simulink model "Ctrl_only"  (R2024a)
settings: Solver=FixedStepDiscrete  StartTime=0.0  StopTime=Inf  FixedStep=0.005  RelTol=1e-3
StopFcn:
  | user_confirmed = true;
  | disp('Gestoppt?!')
  | 
  | % stop(t);
  | % delete(t);
  | 
  | %% Switch to Config Mode
  | %Tc3_AI.sysManager.ActivateConfiguration();
  | %
  | % Tc3_AI.SwitchToConfig('local')
  | %
  | % %save Solution
  | % Tc3_AI.SaveSolution();
  | %
  | % %% Close Aktive VS Instance
  | % Tc3_AI.closeVsInstance();
libraries: slpidlib x1
settings Model: SimulationMode=external  Creator=clemensm  LastModifiedBy=pikronthaler
settings OptimizationCC: LocalBlockOutputs=off
settings RTWCC: Description=TwinCAT GRT Target  SystemTargetFile=TwinCatGrt.tlc  GenCodeOnly=on  GenerateMakefile=off  TemplateMakefile=tcgrt_msbuild.tmf  TargetLang=C++
settings STFCustomTargetCC: TargetLangStandard=C++11 (ISO)  ConcurrentExecutionCompliant=on  CombineOutputUpdateFcns=on  CodeInterfacePackaging=Reusable function  CPPClassGenCompliant=on  GRTInterface=off  GenerateAllocFcn=on  UseToolchainInfoCompliant=off  SystemTargetFile=TwinCatGrt.tlc
settings GRTTargetCC: TargetLangStandard=C++11 (ISO)  ParMdlRefBuildCompliant=off  CompOptLevelCompliant=off  MatFileLogging=off  CodeInterfacePackaging=Reusable function  GenerateAllocFcn=on  UseToolchainInfoCompliant=off  ExtMode=on  ExtModeMexFile=TcExtModeClient  MultiInstanceErrorCode=None

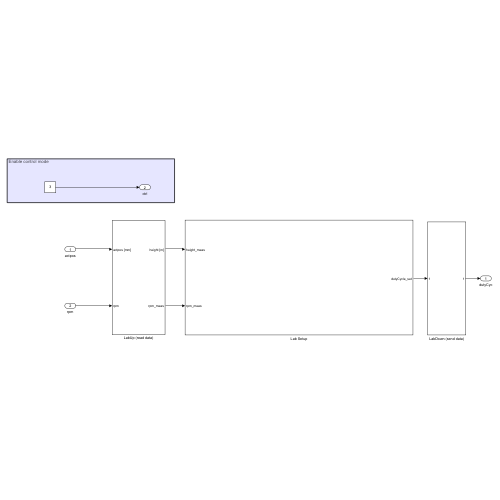
[thumbnail: Simulink's stored preview of the top-level diagram]
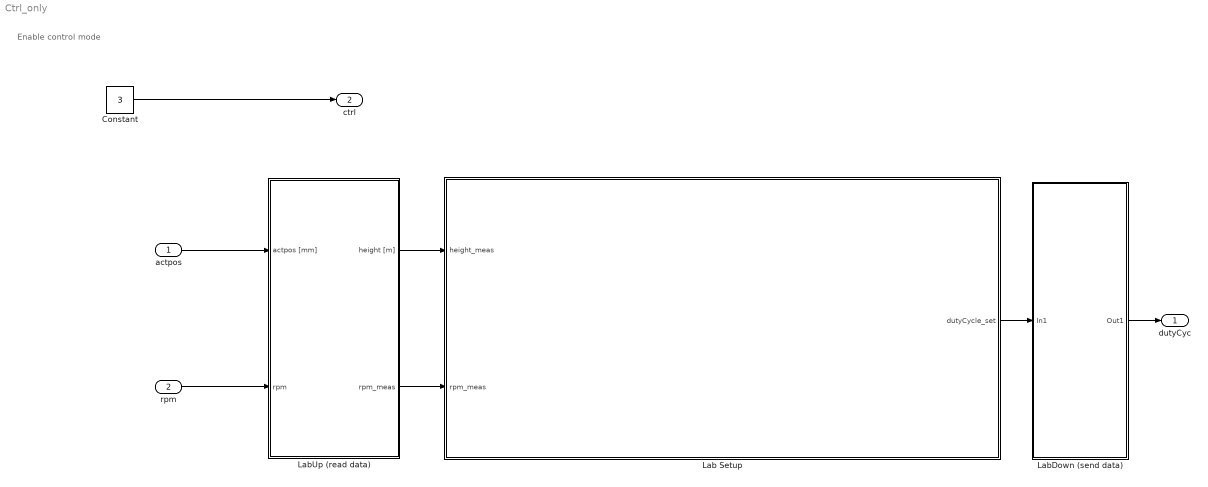
== system Ctrl_only ==
  note: Enable control mode
  actpos : Inport  OutDataTypeStr=uint16
  rpm : Inport  Port=2  OutDataTypeStr=uint16
  Constant : Constant  Value=3  OutDataTypeStr=uint8
  Lab Setup : Subsystem
  LabDown (send data) : Subsystem
  LabUp (read data) : Subsystem
  dutyCyc : Outport  OutDataTypeStr=uint16
  ctrl : Outport  Port=2  OutDataTypeStr=uint8
  wires:
  Constant/1 -> ctrl/1
  LabUp (read data)/2(rpm_meas) -> Lab Setup/2(rpm_meas)
  rpm/1 -> LabUp (read data)/2(rpm)
  LabUp (read data)/1(height [m]) -> Lab Setup/1(height_meas)
  actpos/1 -> LabUp (read data)/1(actpos [mm])
  Lab Setup/1(dutyCycle_set) -> LabDown (send data)/1(In1)
  LabDown (send data)/1(Out1) -> dutyCyc/1

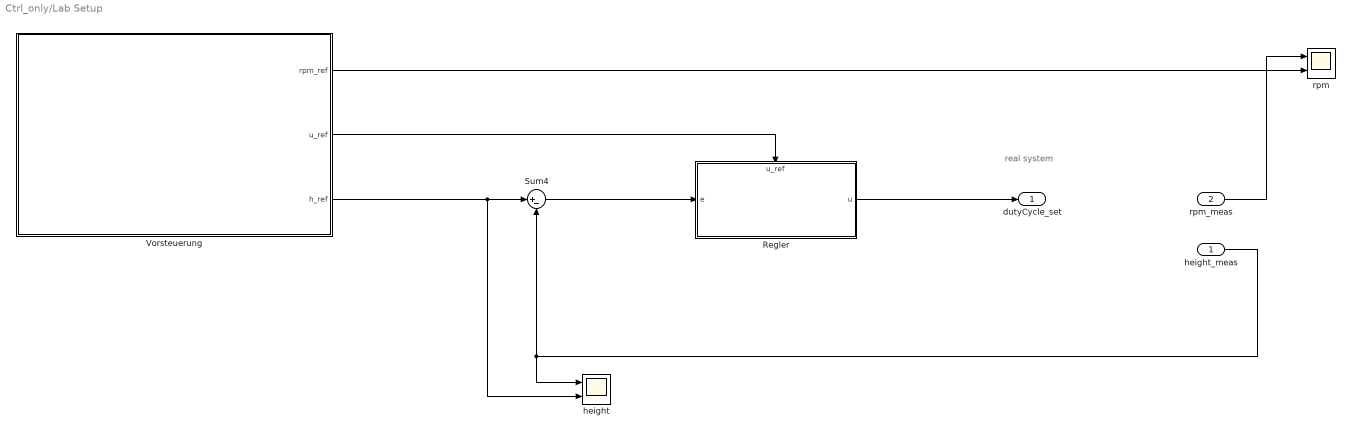
== system Ctrl_only/Lab Setup ==
  note: real system
  height_meas : Inport
  rpm_meas : Inport  Port=2
  Regler : Subsystem
      settings: PortSchema="{\"entries\":[{\"content\":{\"sides\":[{\"content\":{\"connectorIds\":[\"In1\"]},\"type\":\"ConnectorPlacement.EquallySpacedRectSide\",\"uuid\":\"368b1d1f-ffb1-4e6b-b9fe-083329fa83ff\"},{\"content\":{\"connectorIds\":[\"Out1\"],\"side\":\"RIGHT\"},\"type\":\"ConnectorPlacement.EquallySpacedRectSide\",\"uuid\":\"b6a3e5b0-4217-4560-ab72-51db08b1fa5c\"},{\"content\":{\"connectorIds\":[\"In2\"],\"side\":\"TOP\"},\"type\":\"ConnectorPlacement.EquallySpacedRectSide\",\"uuid\":\"ca46bd49-adac-4614-8e8d-04b2e9e52b66\"}]},\"type\":\"ConnectorPlacement.EquallySpacedConnector\",\"uuid\":\"bc9435da-4a52-4305-8584-3547e54afaf1\"}],\"packageUris\":[\"http://schema.mathworks.com/mf0/Connector/R2020b\"],\"version\":\"1.0\"}"
  Sum4 : Sum  Inputs=|+-
  Vorsteuerung : Subsystem
  height : Scope  NumInputPorts=2
  rpm : Scope  NumInputPorts=2
  dutyCycle_set : Outport
  wires:
  height_meas/1 -> Sum4/2, height/1
  rpm_meas/1 -> rpm/1
  Vorsteuerung/3(h_ref) -> height/2, Sum4/1
  Vorsteuerung/1(rpm_ref) -> rpm/2
  Vorsteuerung/2(u_ref) -> Regler/2(u_ref)
  Sum4/1 -> Regler/1(e)
  Regler/1(u) -> dutyCycle_set/1

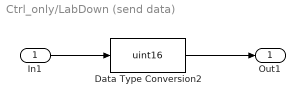
== system Ctrl_only/LabDown (send data) ==
  In1 : Inport
  Data Type Conversion2 : DataTypeConversion  OutDataTypeStr=uint16  SaturateOnIntegerOverflow=off  RndMeth=Floor
  Out1 : Outport
  wires:
  Data Type Conversion2/1 -> Out1/1
  In1/1 -> Data Type Conversion2/1

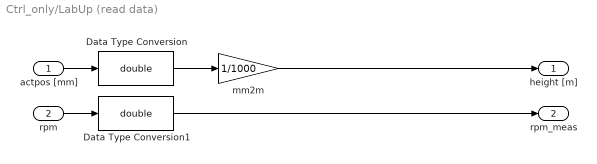
== system Ctrl_only/LabUp (read data) ==
  actpos [mm] : Inport  OutDataTypeStr=uint16
  rpm : Inport  Port=2
  Data Type Conversion : DataTypeConversion  OutDataTypeStr=double  SaturateOnIntegerOverflow=off  RndMeth=Floor
  Data Type Conversion1 : DataTypeConversion  OutDataTypeStr=double  SaturateOnIntegerOverflow=off  RndMeth=Floor
  mm2m : Gain  Gain=1/1000
  height [m] : Outport
  rpm_meas : Outport  Port=2
  wires:
  actpos [mm]/1 -> Data Type Conversion/1
  Data Type Conversion/1 -> mm2m/1
  mm2m/1 -> height [m]/1
  rpm/1 -> Data Type Conversion1/1
  Data Type Conversion1/1 -> rpm_meas/1

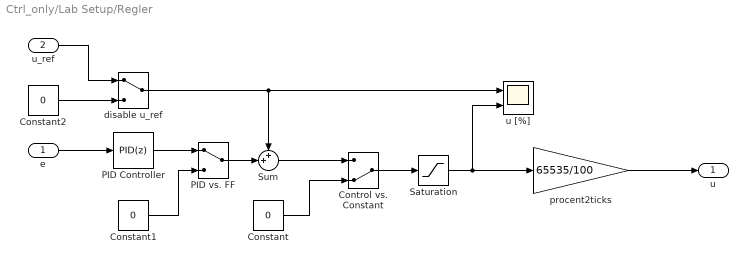
== system Ctrl_only/Lab Setup/Regler ==
  e : Inport
  u_ref : Inport  Port=2
  Constant : Constant  Value=0
  Constant1 : Constant  Value=0
  Constant2 : Constant  Value=0
  Control vs. Constant : ManualSwitch  CurrentSetting=0
  PID Controller : slpidlib/PID Controller  Controller=PID  Form=Parallel  TimeDomain=Discrete-time  UseExternalTs=off  SampleTime=-1  IntegratorMethod=Forward Euler  FilterMethod=Forward Euler  ControllerParametersSource=internal  P=1  I=1  UseKiTs=off  D=0  UseExternalDerivativeSource=off  N=100  UseFilter=on  TunerSelectOption=Transfer Function Based (PID Tuner App)  InitialConditionSource=internal  InitialConditionForIntegrator=0  InitialConditionForFilter=0  DifferentiatorICPrevScaledInput=0  ExternalReset=none  TrackingMode=off  Kt=1  LimitOutput=off  SatLimitsSource=internal  UpperSaturationLimit=inf  LowerSaturationLimit=-inf  LinearizeAsGain=on  AntiWindupMode=none  Kb=1  LimitIntegrator=off  UpperIntegratorSaturationLimit=inf  LowerIntegratorSaturationLimit=-inf  POutMin=[]  POutMax=[]  IOutMin=[]  IOutMax=[]  DOutMin=[]  DOutMax=[]  NOutMin=[]  NOutMax=[]  SumOutMin=[]  SumOutMax=[]  SaturationOutMin=[]  SaturationOutMax=[]  PParamMin=[]  PParamMax=[]  IParamMin=[]  IParamMax=[]  DParamMin=[]  DParamMax=[]  NParamMin=[]  NParamMax=[]  KbParamMin=[]  KbParamMax=[]  KtParamMin=[]  KtParamMax=[]  KbOutMin=[]  KbOutMax=[]  KtOutMin=[]  KtOutMax=[]  IntegratorOutMin=[]  IntegratorOutMax=[]  FilterOutMin=[]  FilterOutMax=[]  SumI1OutMin=[]  SumI1OutMax=[]  SumI2OutMin=[]  SumI2OutMax=[]  SumI3OutMin=[]  SumI3OutMax=[]  SumI4OutMin=[]  SumI4OutMax=[]  SumDOutMin=[]  SumDOutMax=[]  DifferentiatorOutMin=[]  DifferentiatorOutMax=[]  FilterDiffOutCoefMin=[]  FilterDiffOutCoefMax=[]  ReciprocalOutMin=[]  ReciprocalOutMax=[]  SumDenOutMin=[]  SumDenOutMax=[]  SumNumOutMin=[]  SumNumOutMax=[]  DivideOutMin=[]  DivideOutMax=[]  UdiffTsProdOutMin=[]  UdiffTsProdOutMax=[]  NTsProdOutMin=[]  NTsProdOutMax=[]  UintegralTsProdOutMin=[]  UintegralTsProdOutMax=[]  UngainTsProdOutMin=[]  UngainTsProdOutMax=[]  ClampingZeroOutDataTypeStr=Inherit: Inherit via back propagation  ClampingZeroOutMin=[]  ClampingZeroOutMax=[]  FilterDenConstantOutDataTypeStr=Inherit: Inherit via back propagation  FilterDenConstantOutMin=[]  FilterDenConstantOutMax=[]  PCopyOutDataTypeStr=Inherit: Inherit via back propagation  PCopyOutMin=[]  PCopyOutMax=[]  NCopyOutDataTypeStr=Inherit: Inherit via back propagation  NCopyOutMin=[]  NCopyOutMax=[]  IntegratorContinuousStateAttributes=''  IntegratorStateMustResolveToSignalObject=off  IntegratorRTWStateStorageClass=Auto  FilterContinuousStateAttributes=''  FilterStateMustResolveToSignalObject=off  FilterRTWStateStorageClass=Auto  ParallelPVariant=InternalParameters  IdealPVariant=Disabled  IVariant=InternalParameters  DVariant=InternalParameters  IntegratorVariant=Discrete  SatVariant=Disabled  AWVariant=Passthrough  PCopyVariant=Disabled  TRVariant=Disabled  FdbkBlocksVariant=Forward  IdealPFdbkVariant=Disabled  SatFdbkVariant=Disabled  DerivativeFilterVariant=ForwardEulerFilter  NVariant=InternalParameters  NCopyVariant=Disabled  FilterICVariant=InternalICsFilter  IntegratorICVariant=InternalICs  ExternalResetVariant=Disabled  TRSumVariant=Passthrough  SumFdbkVariant=Disabled  SumVariant=Sum_PID  TsampFilterVariant=InternalTs  TsampNgainVariant=Passthrough  TsampIntegralVariant=Disabled_SignalSpec  ExternalSaturationOutDataTypeStr=Inherit: Same as second input  DerivativeSourceVariant=ErrorSignal
  PID vs. FF : ManualSwitch
  Saturation : Saturate  UpperLimit=100  LowerLimit=0
  Sum : Sum  Inputs=++|
  disable u_ref : ManualSwitch
  procent2ticks : Gain  Gain=65535/100
  u [%] : Scope  NumInputPorts=2
  u : Outport
  wires:
  Saturation/1 -> u [%]/2, procent2ticks/1
  Constant/1 -> Control vs. Constant/2
  procent2ticks/1 -> u/1
  Sum/1 -> Control vs. Constant/1
  Control vs. Constant/1 -> Saturation/1
  disable u_ref/1 -> Sum/1, u [%]/1
  PID vs. FF/1 -> Sum/2
  e/1 -> PID Controller/1
  PID Controller/1 -> PID vs. FF/1
  Constant1/1 -> PID vs. FF/2
  Constant2/1 -> disable u_ref/2
  u_ref/1 -> disable u_ref/1

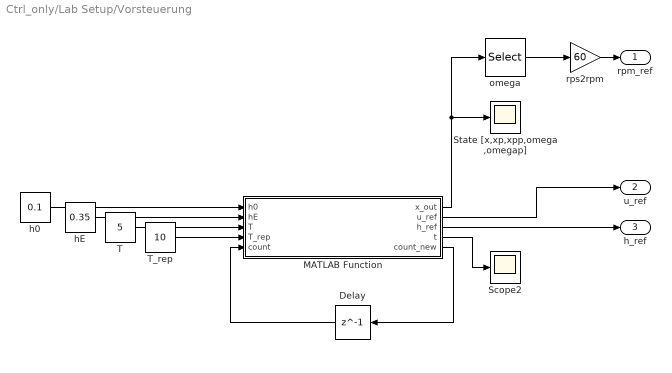
== system Ctrl_only/Lab Setup/Vorsteuerung ==
  Delay : Delay  DelayLength=1
  MATLAB Function : MATLAB Function  TreatAsAtomicUnit=on
  Scope2 : Scope
  State [x,xp,xpp,omega,omegap] : Scope
  T : Constant  Value=5
  T_rep : Constant  Value=10
  h0 : Constant  Value=0.1
  hE : Constant  Value=0.35
  omega : Selector  InputPortWidth=5  IndexOptions=Index vector (dialog)  Indices=4  OutputSizes=1
  rps2rpm : Gain  Gain=60
  rpm_ref : Outport
  u_ref : Outport  Port=2
  h_ref : Outport  Port=3
  wires:
  T/1 -> MATLAB Function/3(T)
  T_rep/1 -> MATLAB Function/4(T_rep)
  h0/1 -> MATLAB Function/1(h0)
  MATLAB Function/1(x_out) -> State [x,xp,xpp,omega,omegap]/1, omega/1
  MATLAB Function/4(t) -> Scope2/1
  hE/1 -> MATLAB Function/2(hE)
  MATLAB Function/5(count_new) -> Delay/1
  omega/1 -> rps2rpm/1
  Delay/1 -> MATLAB Function/5(count)
  MATLAB Function/2(u_ref) -> u_ref/1
  rps2rpm/1 -> rpm_ref/1
  MATLAB Function/3(h_ref) -> h_ref/1

== matlab function Ctrl_only/Lab Setup/Vorsteuerung/MATLAB Function ==
  data: x_out output; u_ref output; h0 input; hE input; T input; T_rep input; h_ref output; t output; count input; count_new output
function [x_out,u_ref,h_ref,t,count_new] = feed_forward(h0,hE,T,T_rep,count)

count_new = count+1;
dT = 0.005;
t = count_new*dT;

% Parameter
g = 9.81;
% ...

% Calculate Trajectory

xp_ref = 0;
xpp_ref = 0;
xppp_ref = 0;

omega = 0;
omega_p = 0;
u = 0;
h_ref = 0;
u_ref = 0;
x_out = zeros(5,1);
end
